simulink model "nlsysid"  (Simulink 8.6)
settings: Solver=ode45  StartTime=0.0  StopTime=U(end,1)  RelTol=1e-3
values from neighbouring files (symbols this model uses):
  b = .5    (= 0.5)    [nonlinid_pendulum.m]
  h = 0.01    [generate_step.m]    (also in nonlinid_pendulum.m = 0.05)
  x0 = [0;0]    [nonlinid_pendulum.m]
settings Model: Creator=dnieuwenhuizen  LastModifiedBy=dnieuwenhuizen
settings OptimizationCC: BooleanDataType=off  ExpressionDepthLimit=128
settings DebuggingCC: SaveWithParameterizedLinksMsg=none  SignalResolutionControl=TryResolveAllWithWarning  SolverPrmCheckMsg=none  MultiTaskDSMMsg=warning  MultiTaskCondExecSysMsg=none  FcnCallInpInsideContextMsg=EnableAllAsError  StateNameClashWarn=none
settings HardwareCC: ProdBitPerPointer=64  ProdLargestAtomicFloat=Float  ProdIntDivRoundTo=Zero  ProdEndianess=LittleEndian  ProdWordSize=64  ProdHWDeviceType=Intel->x86-64 (Windows64)  TargetUnknown=on
settings GRTTargetCC: GeneratePreprocessorConditionals=Use local settings

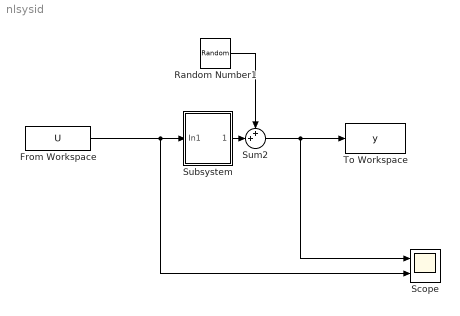
== system nlsysid ==
  From Workspace : FromWorkspace  VariableName=U  SampleTime=h
  Random Number1 : RandomNumber  Variance=1e-5  SampleTime=h
  Scope : Scope  NumInputPorts=2
  Subsystem : Subsystem
  Sum2 : Sum  Inputs=++|  SaturateOnIntegerOverflow=on  InputSameDT=on  OutDataTypeStr=Inherit: Same as first input
  To Workspace : ToWorkspace  VariableName=y  SampleTime=h
  wires:
  From Workspace/1 -> Subsystem/1(In1), Scope/2
  Sum2/1 -> Scope/1, To Workspace/1
  Subsystem/1(Out1) -> Sum2/2
  Random Number1/1 -> Sum2/1

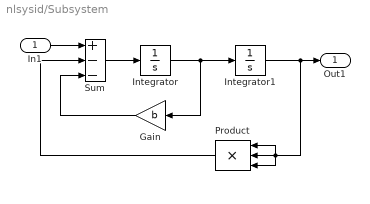
== system nlsysid/Subsystem ==
  In1 : Inport
  Gain : Gain  Gain=b  SaturateOnIntegerOverflow=on  OutDataTypeStr=Inherit: Same as input  ParamDataTypeStr=Inherit: Same as input
  Integrator : Integrator  InitialCondition=x0(2)
  Integrator1 : Integrator  InitialCondition=x0(1)
  Product : Product  Inputs=3  SaturateOnIntegerOverflow=on  RndMeth=Zero  InputSameDT=on  OutDataTypeStr=Inherit: Same as first input
  Sum : Sum  Inputs=+--  SaturateOnIntegerOverflow=on  InputSameDT=on  OutDataTypeStr=Inherit: Same as first input
  Out1 : Outport
  wires:
  Integrator/1 -> Integrator1/1, Gain/1
  Sum/1 -> Integrator/1
  Product/1 -> Sum/2
  Gain/1 -> Sum/3
  In1/1 -> Sum/1
  Integrator1/1 -> Product/2, Product/1, Product/3, Out1/1
